simulink model "findFunction"  (R2024b)
settings: Solver=VariableStepAuto  StartTime=0.0  StopTime=20.0  RelTol=1e-3
libraries: simulink x1
settings Model: Creator=optimus  LastModifiedBy=optimus

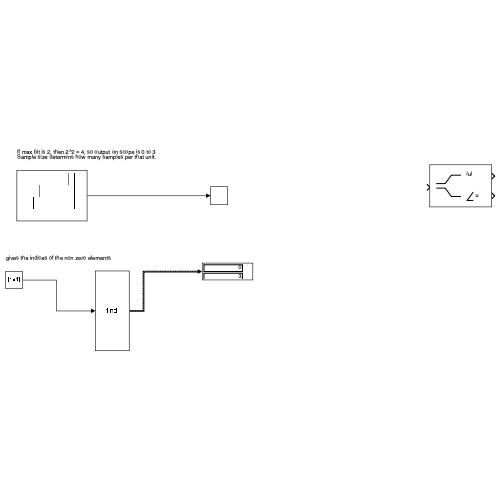
[thumbnail: Simulink's stored preview of the top-level diagram]
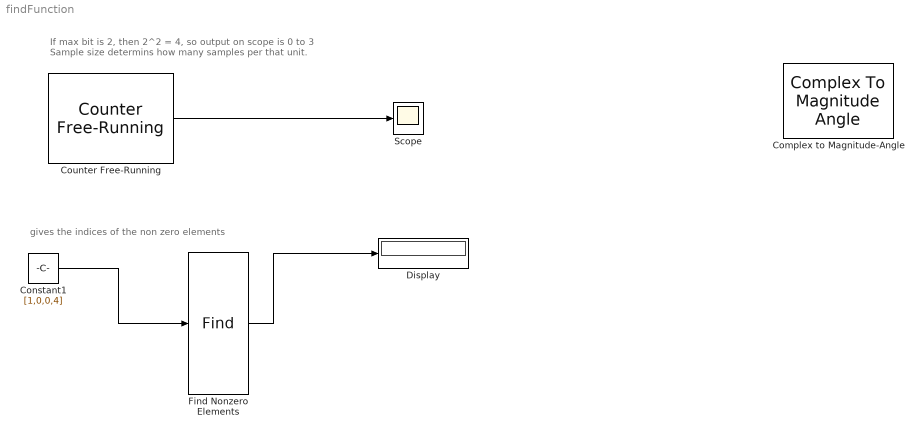
== system findFunction ==
  note: gives the indices of the non zero elements
  note: If max bit is 2, then 2^2 = 4, so output on scope is 0 to 3
      | Sample size determins how many samples per that unit.
  Complex to Magnitude-Angle : ComplexToMagnitudeAngle
  Constant1 : Constant  Value=[1,0,0,4]
  Counter Free-Running : simulink/Sources/Counter Free-Running  NumBits=3  tsamp=1
  Display : Display
  Find Nonzero Elements : Find  NumberOfInputDimensions=1  IndexMode=Zero-based
  Scope : Scope
  wires:
  Counter Free-Running/1 -> Scope/1
  Constant1/1 -> Find Nonzero Elements/1
  Find Nonzero Elements/1 -> Display/1
